simulink model "AngleFilterComponent"  (R2017b)
settings: Solver=FixedStepDiscrete  StartTime=0.0  StopTime=17  FixedStep=0.01  RelTol=1e-3
InitFcn:
  | ra = 4;
  | jm = 0.0000218;
  | rm = 0.7/100;
  | dsm = 62.892;
  | kt = 0.138;
  | ke = kt;
  | ms = 0.93;
  | hl = 1.5 / 100;
  | Lr = 24.1 / 100;
  | Lcm = hl / 2 + Lr;
  | ml =0.182;
  | mr = 0.085;
  | rl = 20.125 / 1000;
  | Jp =1/3 * mr * Lr^2 + 1/2*ml*rl^2 + ml * Lcm ^ 2;
  | Dp = 0.007;
  | g = 9.82;
StartFcn:
  | ra = 4;
  | jm = 0.0000218;
  | rm = 0.7/100;
  | dsm = 62.892;
  | kt = 0.138;
  | ke = kt;
  | ms = 0.93;
libraries: dsparch4 x1
settings Model: Creator=labadmin  LastModifiedBy=labadmin
settings DataIOCC: SaveOutput=off  SaveTime=off
settings RTWCC: SystemTargetFile=sldrt.tlc  TemplateMakefile=sldrt.tmf  Description=Simulink Desktop Real-Time  RTWCompilerOptimization=on
settings CodeAppCC: MaxIdLength=95
settings SimulinkDesktopRealTimeCC: TargetPreCompLibLocation=C:\Program Files\MATLAB\R2017b\toolbox\sldrt\lib\win64

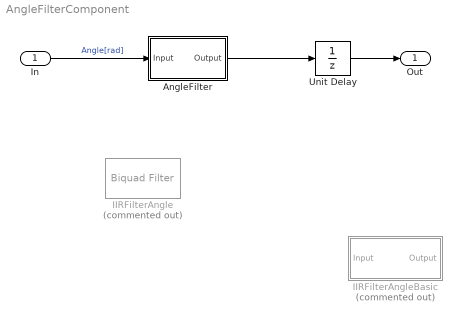
== system AngleFilterComponent ==
  In : Inport  OutDataTypeStr=double  PortDimensions=1  SampleTime=0
  AngleFilter : Subsystem  Tag=FilterWizardSubSystem
      settings: ErrorFcn=dspFilterRealizedInBasicElemsAlgLoopErrFcnCallback
  IIRFilterAngle : dsparch4/Biquad Filter  Tag=BlockMethodSubSystem  Commented=on  IIRFiltStruct=Direct form I  CoeffSource=Specify via dialog  BiQuadCoeffs=[1 2 1 1 -1.7613228110984831 0.804291016029144212;1 1 0 1 -0.802165871687238741 0]  a0Flag=Warning  IC=0  ICnum=0  ICden=0  InputProcessing=Columns as channels (frame based)  denAccumFracLength=30  denProdOutputFracLength=30  secondMemoryFracLength=15  roundingMode=Floor  overflowMode=off  ScaleValues=[0.0107420512326652905;0.0989170641563806297;1]  optimizeScaleValues=on  ScaleValueMode=Specify via input port (g)  scaleValueFracLength=14  FilterSource=Specify via dialog  FilterObject=BQF
      settings: SourceProductName=DSP System Toolbox
  IIRFilterAngleBasic : Subsystem  Tag=FilterWizardSubSystem  Commented=on
      settings: ErrorFcn=dspFilterRealizedInBasicElemsAlgLoopErrFcnCallback
  Unit Delay : UnitDelay  SampleTime=-1
  Out : Outport  OutDataTypeStr=double  PortDimensions=1  SampleTime=[0.01,0]
  wires:
  In/1 -> AngleFilter/1(Input)  "Angle[rad]"
  AngleFilter/1(Output) -> Unit Delay/1
  Unit Delay/1 -> Out/1

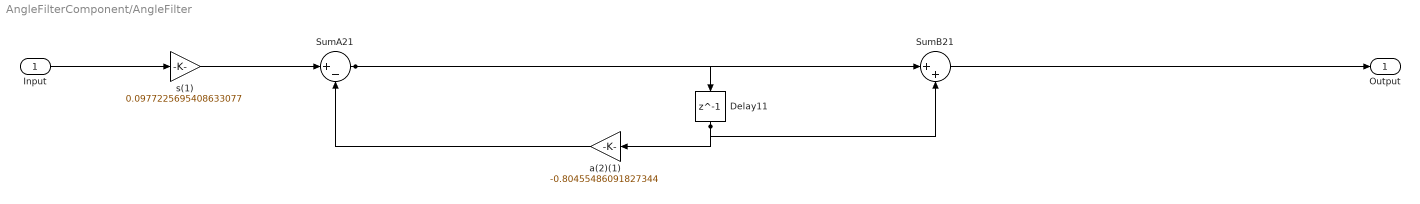
== system AngleFilterComponent/AngleFilter ==
  Input : Inport
  Delay11 : Delay  DelayLength=1  InitialCondition=0
  SumA21 : Sum  Inputs=|+-  RndMeth=Nearest  SaturateOnIntegerOverflow=on  OutDataTypeStr=Inherit: Same as first input
  SumB21 : Sum  Inputs=|++  RndMeth=Nearest  SaturateOnIntegerOverflow=on  OutDataTypeStr=Inherit: Same as first input
  a(2)(1) : Gain  Gain=-0.80455486091827344  ParamDataTypeStr=double  RndMeth=Nearest  SaturateOnIntegerOverflow=on  OutDataTypeStr=Inherit: Same as input
  s(1) : Gain  Gain=0.0977225695408633077  ParamDataTypeStr=double  RndMeth=Nearest  SaturateOnIntegerOverflow=on  OutDataTypeStr=Inherit: Same as input
  Output : Outport
  wires:
  Input/1 -> s(1)/1
  s(1)/1 -> SumA21/1
  SumA21/1 -> SumB21/1, Delay11/1
  SumB21/1 -> Output/1
  a(2)(1)/1 -> SumA21/2
  Delay11/1 -> a(2)(1)/1, SumB21/2

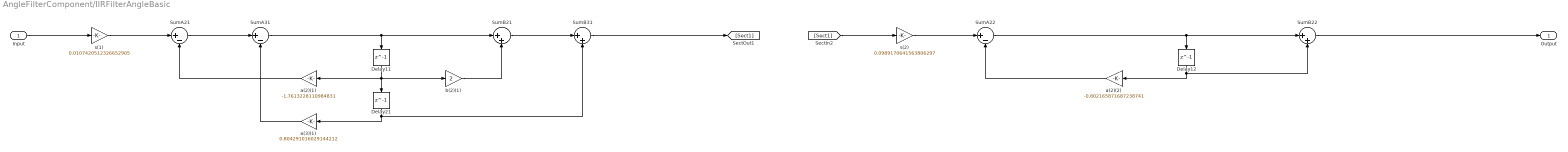
== system AngleFilterComponent/IIRFilterAngleBasic ==
  Input : Inport
  Delay11 : Delay  DelayLength=1  InitialCondition=0
  Delay12 : Delay  DelayLength=1  InitialCondition=0
  Delay21 : Delay  DelayLength=1  InitialCondition=0
  SumA21 : Sum  Inputs=|+-  RndMeth=Nearest  SaturateOnIntegerOverflow=on  OutDataTypeStr=Inherit: Same as first input
  SumA22 : Sum  Inputs=|+-  RndMeth=Nearest  SaturateOnIntegerOverflow=on  OutDataTypeStr=Inherit: Same as first input
  SumA31 : Sum  Inputs=|+-  RndMeth=Nearest  SaturateOnIntegerOverflow=on  OutDataTypeStr=Inherit: Same as first input
  SumB21 : Sum  Inputs=|++  RndMeth=Nearest  SaturateOnIntegerOverflow=on  OutDataTypeStr=Inherit: Same as first input
  SumB22 : Sum  Inputs=|++  RndMeth=Nearest  SaturateOnIntegerOverflow=on  OutDataTypeStr=Inherit: Same as first input
  SumB31 : Sum  Inputs=|++  RndMeth=Nearest  SaturateOnIntegerOverflow=on  OutDataTypeStr=Inherit: Same as first input
  a(2)(1) : Gain  Gain=-1.7613228110984831  ParamDataTypeStr=double  RndMeth=Nearest  SaturateOnIntegerOverflow=on  OutDataTypeStr=Inherit: Same as input
  a(2)(2) : Gain  Gain=-0.802165871687238741  ParamDataTypeStr=double  RndMeth=Nearest  SaturateOnIntegerOverflow=on  OutDataTypeStr=Inherit: Same as input
  a(3)(1) : Gain  Gain=0.804291016029144212  ParamDataTypeStr=double  RndMeth=Nearest  SaturateOnIntegerOverflow=on  OutDataTypeStr=Inherit: Same as input
  b(2)(1) : Gain  Gain=2  ParamDataTypeStr=double  RndMeth=Nearest  SaturateOnIntegerOverflow=on  OutDataTypeStr=Inherit: Same as input
  s(1) : Gain  Gain=0.0107420512326652905  ParamDataTypeStr=double  RndMeth=Nearest  SaturateOnIntegerOverflow=on  OutDataTypeStr=Inherit: Same as input
  s(2) : Gain  Gain=0.0989170641563806297  ParamDataTypeStr=double  RndMeth=Nearest  SaturateOnIntegerOverflow=on  OutDataTypeStr=Inherit: Same as input
  Output : Outport
  wires:
  Input/1 -> s(1)/1
  s(1)/1 -> SumA21/1
  SumA21/1 -> SumA31/1
  SumA31/1 -> SumB21/1, Delay11/1
  SumB21/1 -> SumB31/1
  SumB31/1 -> [Sect1]
  a(2)(1)/1 -> SumA21/2
  Delay11/1 -> a(2)(1)/1, b(2)(1)/1, Delay21/1
  b(2)(1)/1 -> SumB21/2
  a(3)(1)/1 -> SumA31/2
  Delay21/1 -> a(3)(1)/1, SumB31/2
  [Sect1] -> s(2)/1
  s(2)/1 -> SumA22/1
  SumA22/1 -> SumB22/1, Delay12/1
  SumB22/1 -> Output/1
  a(2)(2)/1 -> SumA22/2
  Delay12/1 -> a(2)(2)/1, SumB22/2
